simulink model "building_EXAMPLE_v1"  (R2016b)
settings: Solver=ode23tb  StartTime=-building.preruntime+8760*3600  StopTime=building.runtime+8760*3600  MaxStep=600  EnableMultiTasking=on
StartFcn:
  | tic
StopFcn:
  | toc
values from neighbouring files (symbols this model uses):
  building = create_building_automatic(building, modify, import_mode, name_XML, name_EXCEL, name_PHPP, NUMBEROFZONES)    [work_EXAMPLE_v1.m]
undefined symbols (not defined in the file or in its folder): A, B, C, cp, Dd, Dreifach, FluidMix, get_building, ID, MassFlow, p, Pressure, Qdot_C, Qdot_C_energy, Qdot_H, Qdot_H_energy, Qdot_I_electricity, Qdot_I_electricity_energy, Qdot_I_light, Qdot_I_light_energy, Qdot_I_person, Qdot_I_person_energy, Qdot_S, Qdot_S_energy, Qdot_T_ground, Qdot_T_ground_energy, Qdot_T_neighbour, Qdot_T_neighbour_energy, Qdot_T_opaque, Qdot_T_opaque_energy, Qdot_T_window, Qdot_T_window_energy, Qdot_V_infiltration, Qdot_V_infiltration_energy, Qdot_V_mech, Qdot_V_mech_energy, Qdot_V_window, Qdot_V_window_energy, rho, Tc, Temperature, Tr, Ts, Wärmeschutzglas, x_CO2, x_H2O, x_VOC
libraries: carnotUIBK x1931, carnot x83, simulink_extras x22, simulink x12
(part 1 of 35)
settings Model: SimulationMode=accelerator  Creator=c8461199  LastModifiedBy=eeb
settings SolverCC: ZeroCrossAlgorithm=Adaptive
settings DataIOCC: SaveOutput=off  SignalLogging=off  DSMLogging=off  VisualizeSimOutput=off  SaveTime=off
settings OptimizationCC: UseDivisionForNetSlopeComputation=on  UseFloatMulNetSlope=on  LifeSpan=inf
settings DebuggingCC: MaxConsecutiveZCsMsg=warning  IgnoredZcDiagnostic=none  AllowSymbolicDim=off  SFUnexpectedBacktrackingDiag=warning  SFNoUnconditionalDefaultTransitionDiag=warning  SFExecutionAtInitializationDiag=none
settings ModelReferenceCC: PropagateSignalLabelsOutOfModel=off
settings SFSimCC: SimUserSources=carlib.c
settings RTWCC: BuildConfiguration=Faster Runs
settings GRTTargetCC: TargetLangStandard=C89/C90 (ANSI)
settings ConfigComp: CovMetricSettings=dw  CovHtmlReporting=on  CovSaveCumulativeToWorkspaceVar=on  CovSaveSingleToWorkspaceVar=on  CovExternalEMLEnable=off

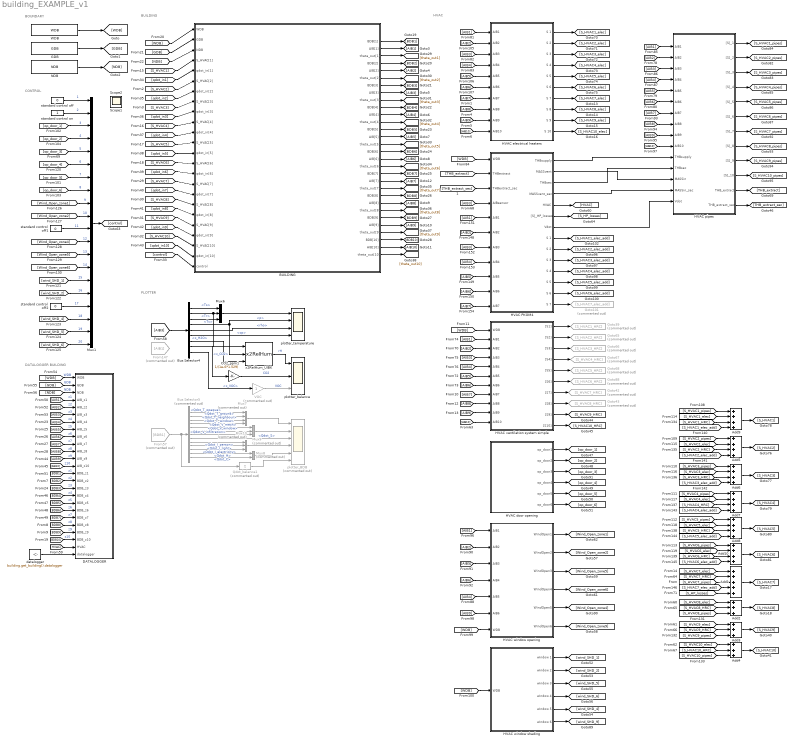
== system building_EXAMPLE_v1 ==
  note: PLOTTER
  note: DATALOGGER BUILDING
  note: BUILDING
  note: BOUNDARY
  note: HVAC
  note: CONTROL
  Add1 : Sum  Inputs=5
  Add{5..10} (6 alike) : Sum  Inputs=4
  Add2 : Sum  Inputs=3
  Add3 : Sum  Inputs=3
  Add4 : Sum  Inputs=3
  BUILDING : Subsystem  mask{building=get_building(building)}
      mask prompts: building "BUILDING object"
      mask init:
      | b = building;
      mask Display:
      | plot(-20,-30,120,100,[10,10,90,90,10],[0,50,50,0,0],...
      |     [100,60,40,0],[40,80,80,40],[20,34,34,20,20],[40,40,20,20,40],...
      |     [60,60,40,40],[0,40,40,0],[65,80,80,65,65],[40,40,20,20,40],...
      |     [47,54,54,47,47],[35,35,4,4,35],[45,41],[20,20])
  Bus Selector4 : BusSelector  OutputSignals=Ts,Tc,Tr,p,rho,cp,x_H2O,x_CO2,x_VOC
  Bus Selector5 : BusSelector  Commented=on  OutputSignals=Qdot_T_opaque,Qdot_T_ground,Qdot_T_neighbour,Qdot_T_window,Qdot_V_mech,Qdot_V_window,Qdot_V_infiltration,Qdot_S,Qdot_I_person,Qdot_I_light,Qdot_I_electricity,Qdot_H,Qdot_C
  CO2_ppm1 : Gain  Gain=1/(1e-6*1.529)
  DATALOGGER : Subsystem
  From147 : From  Commented=on  GotoTag=AIB1
  From57 : From  Commented=on  GotoTag=BDB1
  GDB : carnotUIBK/boundary/GDB  building=get_building(building)
  Goto101 : Goto  Commented=on  GotoTag=S_HVAC7_elec_add
  Goto39 : Goto  Commented=on  GotoTag=S_HVAC1_HRC
  Goto42 : Goto  Commented=on  GotoTag=S_HVAC7_HRC
  Goto43 : Goto  Commented=on  GotoTag=S_HVAC8_HRC
  Goto65 : Goto  Commented=on  GotoTag=S_HVAC2_HRC
  Goto66 : Goto  Commented=on  GotoTag=S_HVAC3_HRC
  Goto67 : Goto  Commented=on  GotoTag=S_HVAC4_HRC
  Goto68 : Goto  Commented=on  GotoTag=S_HVAC5_HRC
  Goto88 : Goto  Commented=on  GotoTag=S_HVAC6_HRC
  HVAC PKOM4 : Subsystem  mask{building=get_building(building), system=7}
      mask init:
      | hvac = building.hvac.get_system(system).parameter;
      mask Display: fprintf('%s',building.hvac.get_system(system).name)
  HVAC door opening : Subsystem  mask{building=get_building(building), system=4}
      mask init:
      | hvac = building.hvac.get_system(system).parameter;
      mask Display: fprintf('%s',building.hvac.get_system(system).name)
  HVAC electrical heaters : Subsystem  mask{building=get_building(building), system=3}
      mask init:
      | hvac = building.hvac.get_system(system).parameter;
      mask Display: fprintf('%s',building.hvac.get_system(system).name)
  HVAC pipes : Subsystem  mask{building=get_building(building), system=9}
      mask init:
      | hvac = building.hvac.get_system(system).parameter;
      mask Display: fprintf('%s',building.hvac.get_system(system).name)
  HVAC ventilation system simple : Subsystem  mask{building=get_building(building), system=8}
      mask init:
      | hvac = building.hvac.get_system(system).parameter;
      mask Display: fprintf('%s',building.hvac.get_system(system).name)
  HVAC window opening : Subsystem  mask{building=get_building(building), system=6}
      mask init:
      | hvac = building.hvac.get_system(system).parameter;
      mask Display: fprintf('%s',building.hvac.get_system(system).name)
  HVAC window shading : Subsystem  mask{building=get_building(building), system=5}
      mask init:
      | hvac = building.hvac.get_system(system).parameter;
      mask Display: fprintf('%s',building.hvac.get_system(system).name)
  Mux1 : Mux  Inputs=[1 1 1 1 1 1 1 1 1 1 1 1 1 1 1 1 1 1 1 1]
  Mux10 : Mux  Commented=on  Inputs=3
  Mux6 : Mux  Inputs=3
  Mux7 : Mux  Commented=on
  Mux8 : Mux  Commented=on  Inputs=2
  Mux9 : Mux  Commented=on  Inputs=3
  NDB : carnotUIBK/boundary/NDB  building=get_building(building)
  Qdot_balance1 : Sum  Commented=on  Inputs=1
  VOC : Gain  Commented=on
  WDB : carnotUIBK/boundary/WDB  building=get_building(building)
  datalogger : Constant  Value=building.get_building().datalogger
  plotter_BDB : Scope  Commented=on  NumInputPorts=6
  plotter_balance : Scope  NumInputPorts=3
  plotter_temperature : Scope  NumInputPorts=4
  standard control off : Constant  Value=0
  standard control off1 : Constant  Value=0
  standard control off2 : Constant  Value=0
  standard control on : Constant
  x2RelHum_UIBK : carnot/Basic/Material_Properties/x2RelHum
  Scope1 : Scope
  Scope2 : Scope
  wires:
  WDB/1 -> [WDB]
  GDB/1 -> [GDB]
  NDB/1 -> [NDB]
  [WDB] -> BUILDING/1(WDB)
  [GDB] -> BUILDING/2(GDB)
  [NDB] -> BUILDING/3(NDB)
  BUILDING/2(AIB[1]) -> [AIB1]
  BUILDING/5(AIB[2]) -> [AIB2]
  BUILDING/8(AIB[3]) -> [AIB3]
  BUILDING/11(AIB[4]) -> [AIB4]
  BUILDING/14(AIB[5]) -> [AIB5]
  BUILDING/17(AIB[6]) -> [AIB6]
  BUILDING/29(AIB[10]) -> [AIB10]
  BUILDING/26(AIB[9]) -> [AIB9]
  BUILDING/23(AIB[8]) -> [AIB8]
  BUILDING/20(AIB[7]) -> [AIB7]
  [S_HVAC5] -> BUILDING/12(S_HVAC[5])
  [S_HVAC4] -> BUILDING/10(S_HVAC[4])
  [S_HVAC1] -> BUILDING/4(S_HVAC[1])
  [S_HVAC2] -> BUILDING/6(S_HVAC[2])
  [S_HVAC3] -> BUILDING/8(S_HVAC[3])
  [S_HVAC6] -> BUILDING/14(S_HVAC[6])
  [S_HVAC10] -> BUILDING/22(S_HVAC[10])
  [S_HVAC9] -> BUILDING/20(S_HVAC[9])
  [S_HVAC8] -> BUILDING/18(S_HVAC[8])
  [S_HVAC7] -> BUILDING/16(S_HVAC[7])
  [control] -> BUILDING/24(control)
  BUILDING/1(BDB[1]) -> [BDB1]
  BUILDING/28(BDB[10]) -> [BDB10]
  BUILDING/4(BDB[2]) -> [BDB2]
  BUILDING/7(BDB[3]) -> [BDB3]
  BUILDING/10(BDB[4]) -> [BDB4]
  BUILDING/13(BDB[5]) -> [BDB5]
  BUILDING/16(BDB[6]) -> [BDB6]
  BUILDING/19(BDB[7]) -> [BDB7]
  BUILDING/22(BDB[8]) -> [BDB8]
  BUILDING/25(BDB[9]) -> [BDB9]
  [qdot_in1] -> BUILDING/5(qdot_in[1])
  [qdot_in9] -> BUILDING/21(qdot_in[9])
  [qdot_in10] -> BUILDING/23(qdot_in[10])
  [qdot_in8] -> BUILDING/19(qdot_in[8])
  [qdot_in7] -> BUILDING/17(qdot_in[7])
  [qdot_in6] -> BUILDING/15(qdot_in[6])
  [qdot_in4] -> BUILDING/11(qdot_in[4])
  [qdot_in5] -> BUILDING/13(qdot_in[5])
  [qdot_in3] -> BUILDING/9(qdot_in[3])
  [qdot_in2] -> BUILDING/7(qdot_in[2])
  BUILDING/3(theta_out[1]) -> [theta_out1]
  BUILDING/30(theta_out[10]) -> [theta_out10]
  BUILDING/27(theta_out[9]) -> [theta_out9]
  BUILDING/24(theta_out[8]) -> [theta_out8]
  BUILDING/21(theta_out[7]) -> [theta_out7]
  BUILDING/18(theta_out[6]) -> [theta_out6]
  BUILDING/15(theta_out[5]) -> [theta_out5]
  BUILDING/12(theta_out[4]) -> [theta_out4]
  BUILDING/9(theta_out[3]) -> [theta_out3]
  BUILDING/6(theta_out[2]) -> [theta_out2]
  datalogger/1 -> DATALOGGER/25(datalogger)
  [AIB1] -> DATALOGGER/4(AIB_z1)  "z1"
  [WDB] -> DATALOGGER/1(WDB)  "WDB"
  [GDB] -> DATALOGGER/2(GDB)  "GDB"
  [NDB] -> DATALOGGER/3(NDB)  "NDB"
  [AIB2] -> DATALOGGER/5(AIB_z2)  "z2"
  [AIB3] -> DATALOGGER/6(AIB_z3)  "z3"
  [AIB4] -> DATALOGGER/7(AIB_z4)  "z4"
  [AIB5] -> DATALOGGER/8(AIB_z5)  "z5"
  [AIB6] -> DATALOGGER/9(AIB_z6)  "z6"
  [AIB7] -> DATALOGGER/10(AIB_z7)  "z7"
  [AIB8] -> DATALOGGER/11(AIB_z8)  "z8"
  [AIB9] -> DATALOGGER/12(AIB_z9)  "z9"
  [AIB10] -> DATALOGGER/13(AIB_z10)  "z10"
  [BDB1] -> DATALOGGER/14(BDB_z1)  "z1"
  [BDB2] -> DATALOGGER/15(BDB_z2)  "z2"
  [BDB3] -> DATALOGGER/16(BDB_z3)  "z3"
  [BDB4] -> DATALOGGER/17(BDB_z4)  "z4"
  [BDB5] -> DATALOGGER/18(BDB_z5)  "z5"
  [BDB6] -> DATALOGGER/19(BDB_z6)  "z6"
  [BDB7] -> DATALOGGER/20(BDB_z7)  "z7"
  [BDB8] -> DATALOGGER/21(BDB_z8)  "z8"
  [BDB9] -> DATALOGGER/22(BDB_z9)  "z9"
  [BDB10] -> DATALOGGER/23(BDB_z10)  "z10"
  Bus Selector4/4 -> x2RelHum_UIBK/2, plotter_temperature/2  "<p>"
  Bus Selector4/1 -> Mux6/1  "<Ts>"
  Bus Selector4/2 -> x2RelHum_UIBK/1, Mux6/2  "<Tc>"
  Bus Selector4/3 -> Mux6/3  "<Tr>"
  Mux6/1 -> plotter_temperature/1
  Bus Selector4/5 -> plotter_temperature/3  "<rho>"
  Bus Selector4/6 -> plotter_temperature/4  "<cp>"
  Bus Selector4/8 -> CO2_ppm1/1  "<x_CO2>"
  Bus Selector4/9 -> VOC/1  "<x_VOC>"
  CO2_ppm1/1 -> plotter_balance/2  "CO2"
  Bus Selector4/7 -> x2RelHum_UIBK/3  "<x_H2O>"
  x2RelHum_UIBK/1 -> plotter_balance/1  "rH"
  Bus Selector5/6 -> Mux9/2  "<Qdot_V_window>"
  Bus Selector5/5 -> Mux9/1  "<Qdot_V_mech>"
  Bus Selector5/4 -> Mux7/4  "<Qdot_T_window>"
  Bus Selector5/3 -> Mux7/3  "<Qdot_T_neighbour>"
  Bus Selector5/2 -> Mux7/2  "<Qdot_T_ground>"
  Bus Selector5/1 -> Mux7/1  "<Qdot_T_opaque>"
  Bus Selector5/7 -> Mux9/3  "<Qdot_V_infiltration>"
  Bus Selector5/8 -> plotter_BDB/3  "<Qdot_S>"
  Bus Selector5/9 -> Mux10/1  "<Qdot_I_person>"
  Bus Selector5/10 -> Mux10/2  "<Qdot_I_light>"
  Bus Selector5/11 -> Mux10/3  "<Qdot_I_electricity>"
  Mux7/1 -> plotter_BDB/1
  From57/1 -> Qdot_balance1/1, Bus Selector5/1
  VOC/1 -> plotter_balance/3  "VOC"
  Mux9/1 -> plotter_BDB/2
  Mux10/1 -> plotter_BDB/4
  Bus Selector5/12 -> Mux8/1  "<Qdot_H>"
  Bus Selector5/13 -> Mux8/2  "<Qdot_C>"
  Mux8/1 -> plotter_BDB/5
  Qdot_balance1/1 -> plotter_BDB/6
  [AIB3] -> Bus Selector4/1
  [HVAC] -> DATALOGGER/24(HVAC)
  [S_HVAC1_pipes] -> Add9/1
  [S_HVAC2_pipes] -> Add5/1
  [S_HVAC3_pipes] -> Add6/1
  [S_HVAC4_pipes] -> Add7/1
  [S_HVAC5_pipes] -> Add8/1
  [S_HVAC6_pipes] -> Add10/1
  [S_HVAC1_elec] -> Add9/2
  [S_HVAC2_elec] -> Add5/2
  [S_HVAC3_elec] -> Add6/2
  [S_HVAC4_elec] -> Add7/2
  [S_HVAC5_elec] -> Add8/2
  [S_HVAC6_elec] -> Add10/2
  Add8/1 -> [S_HVAC5]
  Add7/1 -> [S_HVAC4]
  Add6/1 -> [S_HVAC3]
  Add10/1 -> [S_HVAC6]
  Add9/1 -> [S_HVAC1]
  Add5/1 -> [S_HVAC2]
  [AIB1] -> HVAC electrical heaters/1(AIB1)
  [AIB2] -> HVAC electrical heaters/2(AIB2)
  [AIB3] -> HVAC electrical heaters/3(AIB3)
  [AIB4] -> HVAC electrical heaters/4(AIB4)
  [AIB5] -> HVAC electrical heaters/5(AIB5)
  [AIB6] -> HVAC electrical heaters/6(AIB6)
  HVAC electrical heaters/1(S 1) -> [S_HVAC1_elec]
  HVAC electrical heaters/6(S 6) -> [S_HVAC6_elec]
  HVAC electrical heaters/3(S 3) -> [S_HVAC3_elec]
  HVAC electrical heaters/4(S 4) -> [S_HVAC4_elec]
  HVAC electrical heaters/2(S 2) -> [S_HVAC2_elec]
  HVAC electrical heaters/5(S 5) -> [S_HVAC5_elec]
  HVAC electrical heaters/9(S 9) -> [S_HVAC9_elec]
  HVAC electrical heaters/10(S 10) -> [S_HVAC10_elec]
  HVAC electrical heaters/8(S 8) -> [S_HVAC8_elec]
  HVAC electrical heaters/7(S 7) -> [S_HVAC7_elec]
  [AIB10] -> HVAC electrical heaters/10(AIB10)
  [AIB9] -> HVAC electrical heaters/9(AIB9)
  [AIB8] -> HVAC electrical heaters/8(AIB8)
  [AIB7] -> HVAC electrical heaters/7(AIB7)
  [S_HVAC8_elec] -> Add2/1
  [S_HVAC7_elec] -> Add1/1
  [AIB7] -> HVAC ventilation system simple/8(AIB7)
  [WDB] -> HVAC ventilation system simple/1(WDB)
  HVAC ventilation system simple/7("[S7]") -> Goto42/1
  [AIB8] -> HVAC ventilation system simple/9("AIB8 ")
  [AIB9] -> HVAC ventilation system simple/10(AIB9)
  [AIB10] -> HVAC ventilation system simple/11(AIB10)
  HVAC ventilation system simple/8("[S8]") -> Goto43/1
  HVAC ventilation system simple/9("[S9]") -> [S_HVAC9_HRC]
  HVAC ventilation system simple/10("[S10]") -> [S_HVAC10_HRC]
  Add3/1 -> [S_HVAC9]
  Add1/1 -> [S_HVAC7]
  Add2/1 -> [S_HVAC8]
  Add4/1 -> [S_HVAC10]
  [S_HVAC7_HRC] -> Add1/2
  [S_HVAC8_HRC] -> Add2/2
  [AIB4] -> HVAC pipes/4(AIB4)
  [AIB3] -> HVAC pipes/3(AIB3)
  [AIB2] -> HVAC pipes/2(AIB2)
  [AIB5] -> HVAC pipes/5(AIB5)
  [AIB1] -> HVAC pipes/1(AIB1)
  [AIB6] -> HVAC pipes/6(AIB6)
  HVAC pipes/5("[S]_5") -> [S_HVAC5_pipes]
  HVAC pipes/4("[S]_4") -> [S_HVAC4_pipes]
  HVAC pipes/3("[S]_3") -> [S_HVAC3_pipes]
  HVAC pipes/6("[S]_6") -> [S_HVAC6_pipes]
  HVAC pipes/1("[S]_1") -> [S_HVAC1_pipes]
  HVAC pipes/2("[S]_2") -> [S_HVAC2_pipes]
  HVAC pipes/11(THB_extract) -> [THB_extract]
  [WDB] -> HVAC PKOM4/1(WDB)
  HVAC door opening/1(op_door1) -> [op_door_1]
  HVAC door opening/2(op_door2) -> [op_door_2]
  HVAC door opening/4(op_door4) -> [op_door_4]
  HVAC door opening/5(op_door5) -> [op_door_5]
  HVAC door opening/6(op_door6) -> [op_door_6]
  [AIB3] -> HVAC PKOM4/4(AIBsensor)
  HVAC pipes/12(THB_extract_sec) -> [THB_extract_sec]
  [AIB1] -> HVAC window opening/1(AIB1)
  HVAC window opening/1(WindOpen1) -> [Wind_Open_zone1]
  [AIB2] -> HVAC window opening/2(AIB2)
  [AIB6] -> HVAC window opening/4(AIB4)
  [AIB4] -> HVAC window opening/5(AIB5)
  [AIB9] -> HVAC window opening/6(AIB6)
  HVAC window opening/2(WindOpen2) -> [Wind_Open_zone2]
  HVAC window opening/4(WindOpen4) -> [Wind_Open_zone6]
  HVAC window opening/5(WindOpen5) -> [Wind_Open_zone4]
  HVAC window opening/6(WindOpen6) -> [Wind_Open_zone9]
  [WDB] -> HVAC window opening/7(WDB)
  HVAC PKOM4/5(HVAC) -> [HVAC]
  [WDB] -> HVAC window shading/1(WDB)
  standard control off/1 -> Mux1/1  "1"
  Mux1/1 -> [control]
  standard control on/1 -> Mux1/2  "2"
  [Wind_Open_zone1] -> Mux1/9  "9"
  [Wind_Open_zone6] -> Mux1/14  "14"
  [Wind_Open_zone5] -> Mux1/13  "13"
  [Wind_Open_zone4] -> Mux1/12  "12"
  standard control off1/1 -> Mux1/11  "11"
  [Wind_Open_zone2] -> Mux1/10  "10"
  [op_door_1] -> Mux1/3  "3"
  [op_door_2] -> Mux1/4  "4"
  [op_door_3] -> Mux1/5  "5"
  [op_door_4] -> Mux1/6  "6"
  [op_door_5] -> Mux1/7  "7"
  [op_door_6] -> Mux1/8  "8"
  [wind_SHD_1] -> Mux1/15  "15"
  [wind_SHD_2] -> Mux1/16  "16"
  standard control off2/1 -> Mux1/17  "17"
  [wind_SHD_4] -> Mux1/18  "18"
  [wind_SHD_5] -> Mux1/19  "19"
  [wind_SHD_6] -> Mux1/20  "20"
  HVAC PKOM4/1(THBsupply) -> HVAC pipes/11(THBsupply)
  HVAC PKOM4/2(MASSvent) -> HVAC pipes/13(MASSin)
  HVAC PKOM4/4(MASSvent_sec) -> HVAC pipes/14(MASSin_sec)
  HVAC PKOM4/3(THBsec) -> HVAC pipes/12(THBsec)
  HVAC window shading/2(window 2) -> [wind_SHD_2]
  HVAC window shading/1(window 1) -> [wind_SHD_1]
  HVAC PKOM4/6("[S]_HP_losses") -> [S_HP_losses]
  [THB_extract] -> HVAC PKOM4/2(THBextract)
  [THB_extract_sec] -> HVAC PKOM4/3(THBextract_sec)
  HVAC ventilation system simple/1("[S1]") -> Goto39/1
  HVAC ventilation system simple/2("[S2]") -> Goto65/1
  HVAC ventilation system simple/3("[S3]") -> Goto66/1
  HVAC ventilation system simple/4("[S4]") -> Goto67/1
  HVAC ventilation system simple/5("[S5]") -> Goto68/1
  HVAC ventilation system simple/6("[S6]") -> Goto88/1
  [AIB6] -> HVAC ventilation system simple/7(AIB6)
  [AIB5] -> HVAC ventilation system simple/6(AIB5)
  [AIB4] -> HVAC ventilation system simple/5(AIB4)
  [AIB3] -> HVAC ventilation system simple/4(AIB3)
  [AIB2] -> HVAC ventilation system simple/3(AIB2)
  [AIB1] -> HVAC ventilation system simple/2(AIB1)
  HVAC window shading/3(window 3) -> [wind_SHD_5]
  HVAC window shading/4(window 4) -> [wind_SHD_6]
  HVAC window shading/5(window 5) -> [wind_SHD_4]
  HVAC window shading/6(window 6) -> [wind_SHD_9]
  [AIB5] -> HVAC window opening/3(AIB3)
  HVAC window opening/3(WindOpen3) -> [Wind_Open_zone5]
  HVAC door opening/3(op_door3) -> [op_door_3]
  HVAC pipes/8("[S]_8") -> [S_HVAC8_pipes]
  HVAC pipes/7("[S]_7") -> [S_HVAC7_pipes]
  HVAC pipes/9("[S]_9") -> [S_HVAC9_pipes]
  HVAC pipes/10("[S]_10") -> [S_HVAC10_pipes]
  HVAC PKOM4/7(Vdot) -> HVAC pipes/15(Vdot)
  [AIB7] -> HVAC pipes/7(AIB7)
  [AIB8] -> HVAC pipes/8(AIB8)
  [AIB9] -> HVAC pipes/9(AIB9)
  [AIB10] -> HVAC pipes/10(AIB10)
  [S_HP_losses] -> Add1/5
  [S_HVAC10_HRC] -> Add4/2
  [S_HVAC10_elec] -> Add4/1
  [S_HVAC9_HRC] -> Add3/2
  [S_HVAC9_elec] -> Add3/1
  [S_HVAC8_pipes] -> Add2/3
  [S_HVAC9_pipes] -> Add3/3
  [S_HVAC10_pipes] -> Add4/3
  [S_HVAC2_HRC] -> Add5/3
  [S_HVAC1_HRC] -> Add9/3
  [S_HVAC3_HRC] -> Add6/3
  [S_HVAC4_HRC] -> Add7/3
  [S_HVAC5_HRC] -> Add8/3
  [S_HVAC6_HRC] -> Add10/3
  [S_HVAC1_elec_add] -> Add9/4
  [S_HVAC7_elec_add] -> Add1/4
  [S_HVAC7_pipes] -> Add1/3
  [S_HVAC2_elec_add] -> Add5/4
  [S_HVAC3_elec_add] -> Add6/4
  [S_HVAC4_elec_add] -> Add7/4
  [S_HVAC5_elec_add] -> Add8/4
  [S_HVAC6_elec_add] -> Add10/4
  [AIB7] -> HVAC PKOM4/11(AIB7)
  [AIB6] -> HVAC PKOM4/10(AIB6)
  [AIB5] -> HVAC PKOM4/9(AIB5)
  [AIB4] -> HVAC PKOM4/8(AIB4)
  [AIB3] -> HVAC PKOM4/7(AIB3)
  [AIB2] -> HVAC PKOM4/6(AIB2)
  [AIB1] -> HVAC PKOM4/5(AIB1)
  HVAC PKOM4/8(S 1) -> [S_HVAC1_elec_add]
  HVAC PKOM4/9(S 2) -> [S_HVAC2_elec_add]
  HVAC PKOM4/10(S 3) -> [S_HVAC3_elec_add]
  HVAC PKOM4/11(S 4) -> [S_HVAC4_elec_add]
  HVAC PKOM4/14(S 7) -> Goto101/1
  HVAC PKOM4/13(S 6) -> [S_HVAC6_elec_add]
  HVAC PKOM4/12(S 5) -> [S_HVAC5_elec_add]
